simulink model "DSimulator_abbIRB4HP_OpPIDAda"  (R2021b)
settings: Solver=ode1  StartTime=0.0  StopTime=75  FixedStep=0.001  RelTol=1e-3  EnableMultiTasking=on
values from neighbouring files (symbols this model uses):
  g = 9.81    [run_abb_irb120_OpPIDAda.m]
undefined symbols (not defined in the file or in its folder): Dinamic_abbIRB4HP, plotRobotOpAda, Qpr_abbIRB4Op, Sq_abbIRB4, tauAdaptivePIDR, thetaHatDot_abbIRB4, trajGen_abbIRB4Op, Yr_abbIRB4
CloseFcn:
  | EraseHandles
Description:
  | This model simualtes the robot ABB IRB-120 (4DOF) with a P(I)D-like controller with robot regressor.
settings Model: Creator=E. Dean  LastModifiedBy=dean
settings SolverCC: ConcurrentTasks=on  AlgebraicLoopSolver=TrustRegion
settings DataIOCC: LimitDataPoints=on  SaveFormat=Array  SignalLoggingSaveFormat=ModelDataLogs  ReturnWorkspaceOutputs=off
settings OptimizationCC: ExpressionDepthLimit=2147483647  LifeSpan=inf
settings DebuggingCC: UnderspecifiedInitializationDetection=Classic  MergeDetectMultiDrivingBlocksExec=none  SolverPrmCheckMsg=warning  FcnCallInpInsideContextMsg=warning  StateNameClashWarn=warning  SFUnexpectedBacktrackingDiag=warning  SFNoUnconditionalDefaultTransitionDiag=warning  SFExecutionAtInitializationDiag=none  SFMachineParentedDataDiag=warning  ArithmeticOperatorsInVariantConditions=warning
settings HardwareCC: ProdBitPerPointer=32  ProdBitPerSizeT=32  ProdBitPerPtrDiffT=32  ProdLargestAtomicFloat=None  ProdIntDivRoundTo=Undefined  ProdEndianess=Unspecified  ProdWordSize=32  ProdHWDeviceType=32-bit Generic
settings ModelReferenceCC: PropagateSignalLabelsOutOfModel=off
settings SFSimCC: SimUseLocalCustomCode=off  CustomCodeUndefinedFunction=UseInterfaceOnly
settings RTWCC: RTWUseLocalCustomCode=off
settings CodeAppCC: StateflowObjectComments=on
settings GRTTargetCC: TargetLangStandard=C89/C90 (ANSI)  CombineOutputUpdateFcns=off  GRTInterface=on
settings ConfigComp: CovMetricSettings=dw  CovSaveCumulativeToWorkspaceVar=on  CovSaveSingleToWorkspaceVar=on

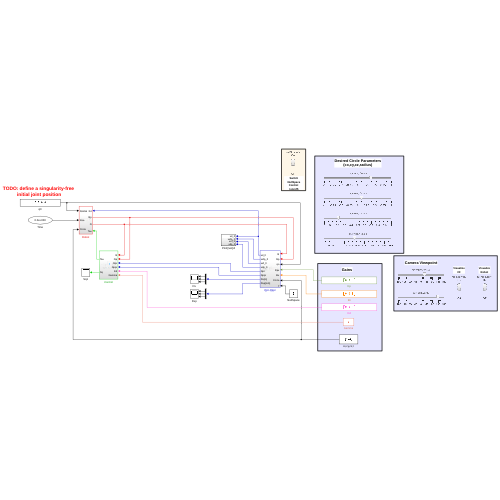
[thumbnail: Simulink's stored preview of the top-level diagram]
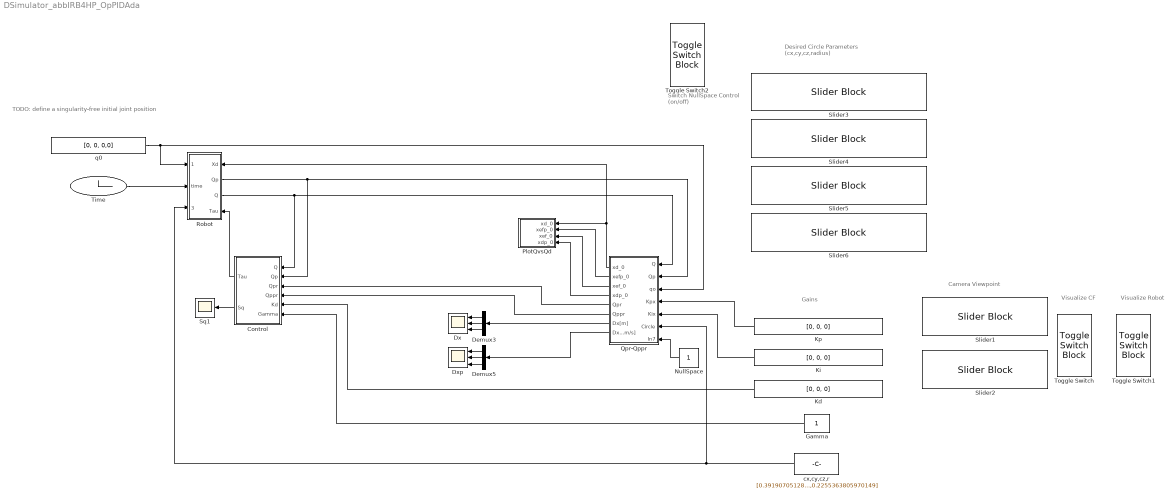
== system DSimulator_abbIRB4HP_OpPIDAda ==
  note: TODO: define a singularity-free
      | initial joint position
  note: Gains
  note: Visualize
      | CF
  note: Desired Circle Parameters
      | (cx,cy,cz,radius)
  note: Camera Viewpoint
  note: Visualize
      | Robot
  note: Switch
      | NullSpace
      | Control
      | (on/off)
  Control : Subsystem
  Demux3 : Demux  Outputs=3
  Demux5 : Demux  Outputs=3
  Dx : Scope  NumInputPorts=3
  Dxp : Scope  NumInputPorts=3
  Gamma : Constant
  Kd : Constant  Value=[0, 0, 0]
  Ki : Constant  Value=[0, 0, 0]
  Kp : Constant  Value=[0, 0, 0]
  NullSpace : Constant
  PlotQvsQd : Subsystem
  Qpr-Qppr : Subsystem
  Robot : Subsystem
      settings: PortSchema="{\"entries\":[{\"content\":{\"sides\":[{\"content\":{\"connectorIds\":[\"In1\",\"In2\",\"In3\"]},\"type\":\"ConnectorPlacement.EquallySpacedRectSide\",\"uuid\":\"6d5847ae-86f7-4e83-b011-f9e0bdbf9fe5\"},{\"content\":{\"connectorIds\":[\"In4\",\"Out1\",\"Out2\",\"In5\"],\"side\":\"RIGHT\"},\"type\":\"ConnectorPlacement.EquallySpacedRectSide\",\"uuid\":\"f4b7c6cc-ce44-45e7-a236-775b672f12f1\"},{\"content\":{\"connectorIds\":[],\"side\":\"TOP\"},\"type\":\"ConnectorPlacement.EquallySpacedRectSide\",\"uuid\":\"c0c3f5b0-9276-4138-918b-c147d2796a8f\"}]},\"type\":\"ConnectorPlacement.EquallySpacedConnector\",\"uuid\":\"473e7ef7-70e2-41c1-b4cb-255091f4b29f\"}],\"packageUris\":[\"http://schema.mathworks.com/mf0/Connector/R2020b\"],\"version\":\"1.0\"}"
  Slider1 : SliderBlock  ScaleMin=-180  ScaleMax=180  TickInterval=45
  Slider2 : SliderBlock  ScaleMin=-180  ScaleMax=180  TickInterval=45
  Slider3 : SliderBlock  ScaleMin=-1  ScaleMax=1  TickInterval=0.25
  Slider4 : SliderBlock  ScaleMin=-1  ScaleMax=1  TickInterval=0.25
  Slider5 : SliderBlock  ScaleMax=1  TickInterval=0.1
  Slider6 : SliderBlock  ScaleMax=0.5  TickInterval=0.05
  Sq1 : Scope
  Time : Clock
  Toggle Switch : ToggleSwitchBlock
      settings: Values={{'Off', 'On'}, [0 1]}
  Toggle Switch1 : ToggleSwitchBlock
      settings: Values={{'Off', 'On'}, [0 1]}
  Toggle Switch2 : ToggleSwitchBlock
      settings: Values={{'Off', 'On'}, [0 1]}
  cx,cy,cz,r : Constant  Value=[0.3919070512820513,0.104727564102564,0.204,0.2255363805970149]
  q0 : Constant  Value=[0, 0, 0,0]
  wires:
  Demux3/2 -> Dx/2
  Demux3/1 -> Dx/1
  Demux3/3 -> Dx/3
  Kd/1 -> Control/5(Kd)
  Demux5/1 -> Dxp/1
  Demux5/3 -> Dxp/3
  Demux5/2 -> Dxp/2
  Kp/1 -> Qpr-Qppr/4(Kpx)
  Ki/1 -> Qpr-Qppr/5(Kix)
  Qpr-Qppr/7(Dx[m]) -> Demux3/1
  Qpr-Qppr/8(Dxp[m/s]) -> Demux5/1
  Qpr-Qppr/1(xd_0) -> Robot/4(Xd), PlotQvsQd/1(xd_0)
  Qpr-Qppr/4(xdp_0) -> PlotQvsQd/4(xdp_0)
  Qpr-Qppr/5(Qpr) -> Control/3(Qpr)
  Qpr-Qppr/6(Qppr) -> Control/4(Qppr)
  Control/2(Sq) -> Sq1/1
  Robot/2(Q) -> Qpr-Qppr/1(Q), Control/1(Q)
  Robot/1(Qp) -> Control/2(Qp), Qpr-Qppr/2(Qp)
  q0/1 -> Robot/1(Qinitial), Qpr-Qppr/3(qo)
  Time/1 -> Robot/2(time)
  Control/1(Tau) -> Robot/5(Tau)
  Gamma/1 -> Control/6(Gamma)
  Qpr-Qppr/3(xef_0) -> PlotQvsQd/3(xef_0)
  Qpr-Qppr/2(xefp_0) -> PlotQvsQd/2(xefp_0)
  cx,cy,cz,r/1 -> Qpr-Qppr/6(Circle), Robot/3(Circle)
  NullSpace/1 -> Qpr-Qppr/7(In7)

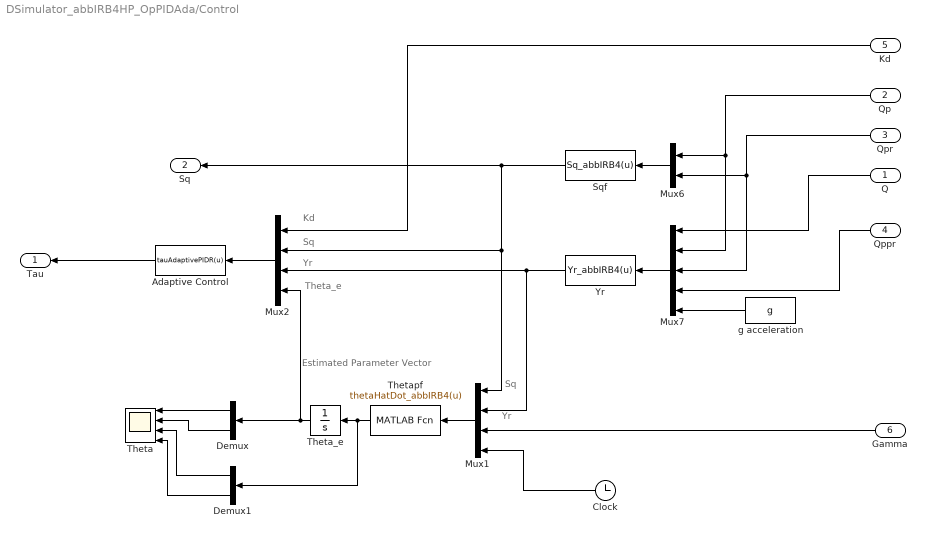
== system DSimulator_abbIRB4HP_OpPIDAda/Control ==
  note: Theta_e
  note: Estimated
      | Parameter
      | Vector
  note: Yr
  note: Sq
  note: Kd
  note: Yr
  note: Sq
  Q : Inport
  Qp : Inport  Port=2
  Qpr : Inport  Port=3
  Qppr : Inport  Port=4
  Kd : Inport  Port=5
  Gamma : Inport  Port=6
  Adaptive Control : MATLABFcn  MATLABFcn=tauAdaptivePIDR(u)  OutputDimensions=4
  Clock : Clock
  Demux : Demux  Outputs=2
  Demux1 : Demux  Outputs=2
  Mux1 : Mux
  Mux2 : Mux
  Mux6 : Mux  Inputs=2
  Mux7 : Mux  Inputs=5
  Sqf : MATLABFcn  MATLABFcn=Sq_abbIRB4(u)  OutputDimensions=4
  Theta : Scope  NumInputPorts=4
  Theta_e : Integrator
  Thetapf : MATLABFcn  MATLABFcn=thetaHatDot_abbIRB4(u)  OutputDimensions=39
  Yr : MATLABFcn  MATLABFcn=Yr_abbIRB4(u)  OutputDimensions=4*39
  g acceleration : Constant  Value=g
  Tau : Outport
  Sq : Outport  Port=2
  wires:
  Yr/1 -> Mux1/2, Mux2/3
  g acceleration/1 -> Mux7/5
  Qpr/1 -> Mux7/3, Mux6/2
  Qppr/1 -> Mux7/4
  Mux7/1 -> Yr/1
  Mux6/1 -> Sqf/1
  Mux2/1 -> Adaptive Control/1
  Qp/1 -> Mux7/2, Mux6/1
  Kd/1 -> Mux2/1
  Adaptive Control/1 -> Tau/1
  Q/1 -> Mux7/1
  Sqf/1 -> Sq/1, Mux2/2, Mux1/1
  Mux1/1 -> Thetapf/1
  Gamma/1 -> Mux1/3
  Clock/1 -> Mux1/4
  Thetapf/1 -> Demux1/1, Theta_e/1
  Theta_e/1 -> Demux/1, Mux2/4
  Demux/1 -> Theta/1
  Demux/2 -> Theta/2
  Demux1/1 -> Theta/3
  Demux1/2 -> Theta/4

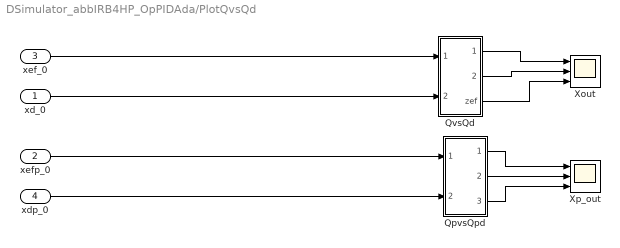
== system DSimulator_abbIRB4HP_OpPIDAda/PlotQvsQd ==
  xd_0 : Inport
  xefp_0 : Inport  Port=2
  xef_0 : Inport  Port=3
  xdp_0 : Inport  Port=4
  QpvsQpd : Subsystem
  QvsQd : Subsystem
  Xout : Scope  NumInputPorts=3
  Xp_out : Scope  NumInputPorts=3
  wires:
  QvsQd/2(yef) -> Xout/2
  QvsQd/3(zef) -> Xout/3
  QpvsQpd/2(ypo) -> Xp_out/2
  xef_0/1 -> QvsQd/1(xef_0)
  xefp_0/1 -> QpvsQpd/1(xefp_0)
  QpvsQpd/3(zpo) -> Xp_out/3
  xd_0/1 -> QvsQd/2(xd_0)
  QpvsQpd/1(xpo) -> Xp_out/1
  QvsQd/1(xef) -> Xout/1
  xdp_0/1 -> QpvsQpd/2(xdp_0)

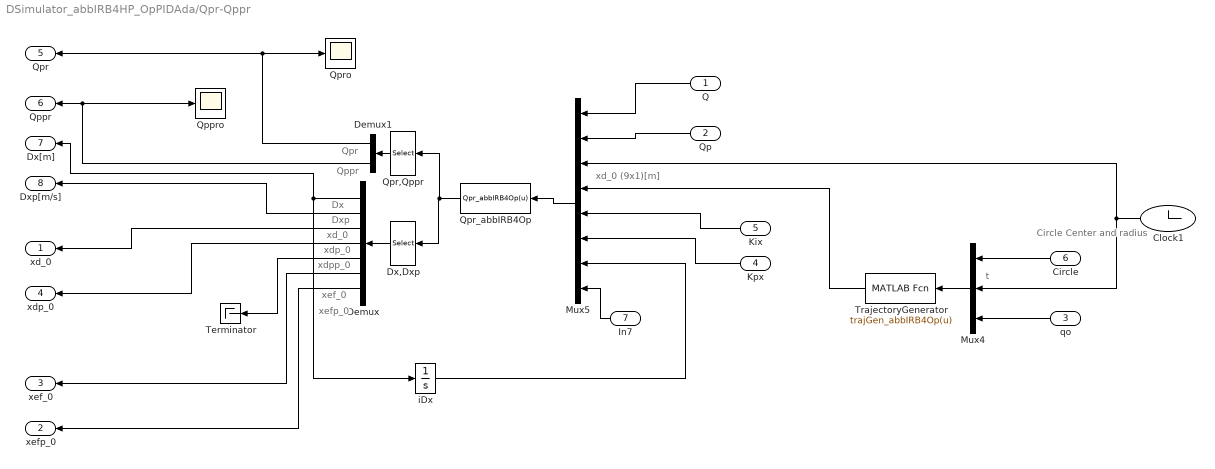
== system DSimulator_abbIRB4HP_OpPIDAda/Qpr-Qppr ==
  note: xef_0
  note: Circle Center
      | and radius
  note: xdpp_0
  note: Qpr
  note: t
  note: xd_0 (9x1)[m]
  note: Dx
  note: Dxp
  note: xd_0
  note: xdp_0
  note: Qppr
  note: xefp_0
  Q : Inport
  Qp : Inport  Port=2
  qo : Inport  Port=3
  Kpx : Inport  Port=4
  Kix : Inport  Port=5
  Circle : Inport  Port=6
  In7 : Inport  Port=7
  Clock1 : Clock
  Demux : Demux  Outputs=7
  Demux1 : Demux  Outputs=2
  Dx,Dxp : Selector  InputPortWidth=29  IndexOptions=Index vector (dialog)  Indices=[9:29]  OutputSizes=1
  Mux4 : Mux  Inputs=3
  Mux5 : Mux  Inputs=8
  Qppro : Scope
  Qpr,Qppr : Selector  InputPortWidth=29  IndexOptions=Index vector (dialog)  Indices=[1:8]  OutputSizes=1
  Qpr_abbIRB4Op : MATLABFcn  MATLABFcn=Qpr_abbIRB4Op(u)  OutputDimensions=29
  Qpro : Scope
  Terminator : Terminator
  TrajectoryGenerator : MATLABFcn  MATLABFcn=trajGen_abbIRB4Op(u)  OutputDimensions=9
  iDx : Integrator
  xd_0 : Outport
  xefp_0 : Outport  Port=2
  xef_0 : Outport  Port=3
  xdp_0 : Outport  Port=4
  Qpr : Outport  Port=5
  Qppr : Outport  Port=6
  Dx[m] : Outport  Port=7
  Dxp[m/s] : Outport  Port=8
  wires:
  Mux4/1 -> TrajectoryGenerator/1
  Mux5/1 -> Qpr_abbIRB4Op/1
  Demux/5 -> Terminator/1
  iDx/1 -> Mux5/7
  Demux/2 -> Dxp[m/s]/1
  Kix/1 -> Mux5/5
  Demux/1 -> Dx[m]/1, iDx/1
  Demux1/1 -> Qpro/1, Qpr/1
  Kpx/1 -> Mux5/6
  Qp/1 -> Mux5/2
  Q/1 -> Mux5/1
  Demux1/2 -> Qppro/1, Qppr/1
  Qpr_abbIRB4Op/1 -> Qpr,Qppr/1, Dx,Dxp/1
  Clock1/1 -> Mux5/3, Mux4/2
  TrajectoryGenerator/1 -> Mux5/4
  Demux/3 -> xd_0/1
  Demux/4 -> xdp_0/1
  Circle/1 -> Mux4/1
  qo/1 -> Mux4/3
  Dx,Dxp/1 -> Demux/1
  Qpr,Qppr/1 -> Demux1/1
  Demux/7 -> xefp_0/1
  Demux/6 -> xef_0/1
  In7/1 -> Mux5/8

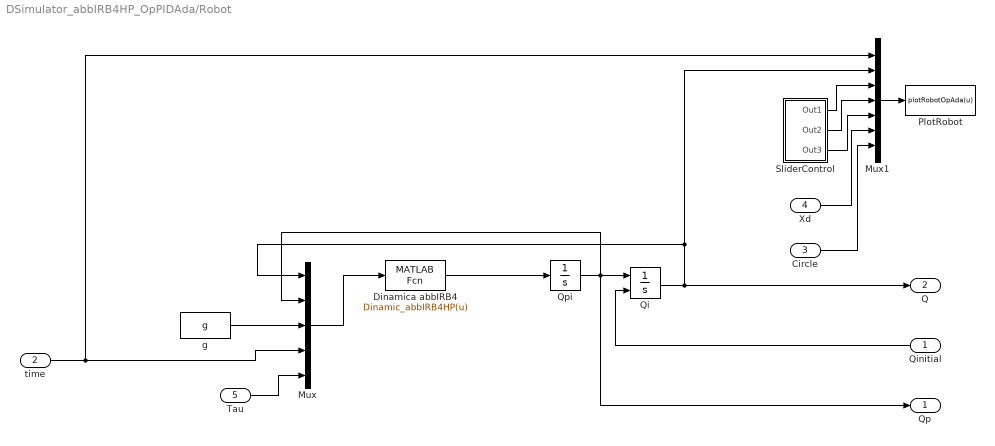
== system DSimulator_abbIRB4HP_OpPIDAda/Robot ==
  Qinitial : Inport
  time : Inport  Port=2
  Circle : Inport  Port=3
  Xd : Inport  Port=4
  Tau : Inport  Port=5
  Dinamica abbIRB4 : MATLABFcn  MATLABFcn=Dinamic_abbIRB4HP(u)  OutputDimensions=4
  Mux : Mux  Inputs=5
  Mux1 : Mux  Inputs=7
  PlotRobot : MATLABFcn  MATLABFcn=plotRobotOpAda(u)  OutputDimensions=0
  Qi : Integrator  InitialConditionSource=external  InitialCondition=[0;0;0;0]
  Qpi : Integrator  InitialCondition=[0;0;0;0]
  SliderControl : Subsystem
  g : Constant  Value=g
  Qp : Outport
  Q : Outport  Port=2
  wires:
  SliderControl/2(Out2) -> Mux1/4
  g/1 -> Mux/3
  Qpi/1 -> Mux/2, Qi/1, Qp/1
  Dinamica abbIRB4/1 -> Qpi/1
  Mux1/1 -> PlotRobot/1
  Mux/1 -> Dinamica abbIRB4/1
  time/1 -> Mux1/1, Mux/4
  Tau/1 -> Mux/5
  Qi/1 -> Q/1, Mux1/2, Mux/1
  Qinitial/1 -> Qi/2
  SliderControl/1(Out1) -> Mux1/3
  SliderControl/3(Out3) -> Mux1/5
  Xd/1 -> Mux1/6
  Circle/1 -> Mux1/7

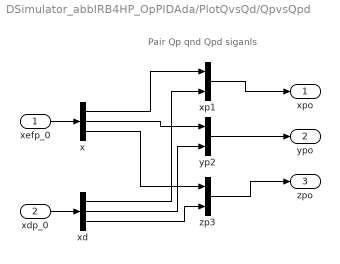
== system DSimulator_abbIRB4HP_OpPIDAda/PlotQvsQd/QpvsQpd ==
  note: Pair Qp qnd Qpd siganls
  xefp_0 : Inport
  xdp_0 : Inport  Port=2
  x : Demux  Outputs=3
  xd : Demux  Outputs=3
  xp1 : Mux  Inputs=2
  yp2 : Mux  Inputs=2
  zp3 : Mux  Inputs=2
  xpo : Outport
  ypo : Outport  Port=2
  zpo : Outport  Port=3
  wires:
  xd/1 -> xp1/2
  xd/2 -> yp2/2
  x/3 -> zp3/1
  x/1 -> xp1/1
  xefp_0/1 -> x/1
  yp2/1 -> ypo/1
  xdp_0/1 -> xd/1
  xp1/1 -> xpo/1
  x/2 -> yp2/1
  zp3/1 -> zpo/1
  xd/3 -> zp3/2

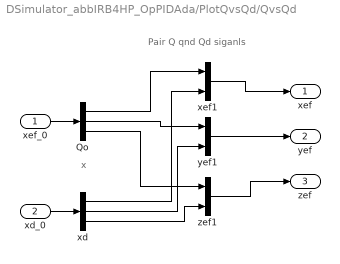
== system DSimulator_abbIRB4HP_OpPIDAda/PlotQvsQd/QvsQd ==
  note: x
  note: Pair Q qnd Qd siganls
  xef_0 : Inport
  xd_0 : Inport  Port=2
  Qo : Demux  Outputs=3
  xd : Demux  Outputs=3
  xef1 : Mux  Inputs=2
  yef1 : Mux  Inputs=2
  zef1 : Mux  Inputs=2
  xef : Outport
  yef : Outport  Port=2
  zef : Outport  Port=3
  wires:
  xd/1 -> xef1/2
  xd/2 -> yef1/2
  Qo/3 -> zef1/1
  Qo/1 -> xef1/1
  xef_0/1 -> Qo/1
  yef1/1 -> yef/1
  xd_0/1 -> xd/1
  xef1/1 -> xef/1
  Qo/2 -> yef1/1
  zef1/1 -> zef/1
  xd/3 -> zef1/2

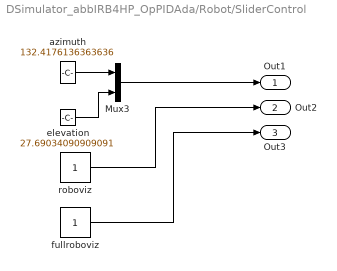
== system DSimulator_abbIRB4HP_OpPIDAda/Robot/SliderControl ==
  Mux3 : Mux  Inputs=2
  azimuth : Constant  Value=132.4176136363636
  elevation : Constant  Value=27.69034090909091
  fullroboviz : Constant
  roboviz : Constant
  Out1 : Outport
  Out2 : Outport  Port=2
  Out3 : Outport  Port=3
  wires:
  azimuth/1 -> Mux3/1
  roboviz/1 -> Out2/1
  elevation/1 -> Mux3/2
  Mux3/1 -> Out1/1
  fullroboviz/1 -> Out3/1
